simulink model "SimCases"  (R2018a)
settings: Solver=FixedStepDiscrete  StartTime=0.0  StopTime=inf  RelTol=1e-3
values from neighbouring files (symbols this model uses):
  Batch = 10    [Main.m]    (also in main.m)
  G_in = [AmbInfo(i,5,2) AmbInfo(i,:,2)]'    [Main.m]    (also in main.m)
  T_in = [AmbInfo(i,5,1) AmbInfo(i,:,1)]'    [Main.m]    (also in main.m)
libraries: dspindex x2, powerlib x1
settings Model: Creator=MATLAB  LastModifiedBy=Clayt-ML
settings OptimizationCC: SimCompilerOptimization=on
settings SFSimCC: SimParseCustomCode=off

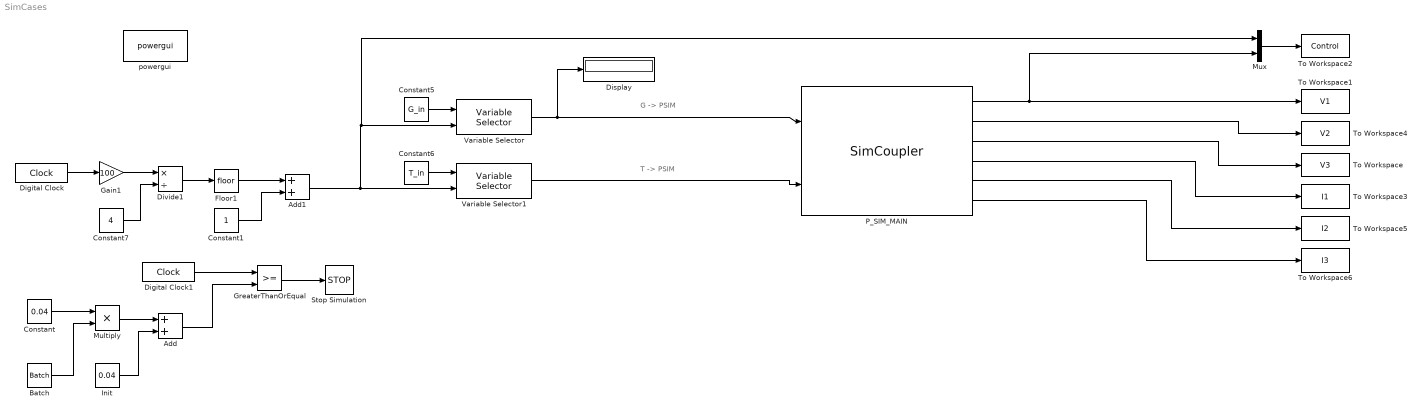
== system SimCases ==
  note: G -> PSIM
  note: T -> PSIM
  Add : Sum
  Add1 : Sum
  Batch : Constant  Value=Batch
  Constant : Constant  Value=0.04
  Constant1 : Constant
  Constant5 : Constant  Value=G_in
  Constant6 : Constant  Value=T_in
  Constant7 : Constant  Value=4
  Digital Clock : DigitalClock  SampleTime=2e-5
  Digital Clock1 : DigitalClock  SampleTime=4e-4
  Display : Display
  Divide1 : Product  Inputs=*/
  Floor1 : Rounding
  Gain1 : Gain  Gain=100
  GreaterThanOrEqual : RelationalOperator  OutDataTypeStr=boolean  RndMeth=Simplest
  Init : Constant  Value=0.04
  Multiply : Product
  Mux : Mux  Inputs=2
  P_SIM_MAIN : S-Function  FunctionName=SimCoupler  Parameters='C:\Users\Clayt-ML\Desktop\SIMUs\___Mono-Fault___02-25\S1-Normal\P_SIM_MAIN.psimsch'  SFunctionDeploymentMode=off  EnableBusSupport=off
      mask init:
      | c=[0:10:360]*pi/180;
      | x1=cos(c)*30; y1=sin(c)*30+20;
      | x2=cos(c)*30;y2=sin(c)*30-20;
      settings: OpenFcn=PsimDialog('PSimFileEdt','Value','Parameters');  CloseFcn=close(gcf);
      mask Display: plot(-60,-60,60,60,x1,y1,x2,y2)
  Stop Simulation : Stop
  To Workspace : ToWorkspace  VariableName=V3  SampleTime=-1
  To Workspace1 : ToWorkspace  VariableName=V1  SampleTime=-1
  To Workspace2 : ToWorkspace  VariableName=Control  SampleTime=-1
  To Workspace3 : ToWorkspace  VariableName=I1  SampleTime=-1
  To Workspace4 : ToWorkspace  VariableName=V2  SampleTime=-1
  To Workspace5 : ToWorkspace  VariableName=I2  SampleTime=-1
  To Workspace6 : ToWorkspace  VariableName=I3  SampleTime=-1
  Variable Selector : dspindex/Variable Selector  NumInputs=1  rowsOrCols=Rows  IdxMode=Variable  Elements=[1 3]  ZerOneIdxMode=One-based  errmode=Clip Index  FillMode=on  FillValues=0
  Variable Selector1 : dspindex/Variable Selector  NumInputs=1  rowsOrCols=Rows  IdxMode=Variable  Elements=[1 3]  ZerOneIdxMode=One-based  errmode=Clip Index  FillMode=on  FillValues=0
  powergui : powerlib/powergui  Priority=1  SimulationMode=Discrete  SampleTime=1e-5  frequency=60  Iterations=50  frequencyindice=60  Pbase=100e6  ErrMax=1e-4  UnitsV=kV  UnitsW=MW  buscounter=0  FunctionMessages=off  echomessages=off  EnableUseOfTLC=off  CurrentSourceSwitches=off  DisableSnubberDevices=off  DisableRonSwitches=off  DisableVfSwitches=off  DisplayEquations=off  SolverType=Tustin/Backward Euler (TBE)  Interpol=off  ExternalGateDelay=off  methode=off  Ts=100  x0status=blocks  SPID=on  SwTol=0  HookPort=off  RestoreLinks=warning  ResistiveCurrentMeasurement=off  Frange=[0:2:500]  Ylog=off  Xlog=on  ShowGrid=off  save=off  variable=ZData  structure=0  ZoomFFT=off  StartTime=0.0  cycles=1  DisplayStyle=1  fundamental=60  FreqAxis=off  MaxFrequency=1000  frequencyindicesteady=1  RmsSteady=1  display=off
  wires:
  Mux/1 -> To Workspace2/1
  Constant5/1 -> Variable Selector/1
  Constant6/1 -> Variable Selector1/1
  Divide1/1 -> Floor1/1
  Gain1/1 -> Divide1/1
  Constant7/1 -> Divide1/2
  P_SIM_MAIN/1 -> Mux/2, To Workspace1/1
  GreaterThanOrEqual/1 -> Stop Simulation/1
  Add/1 -> GreaterThanOrEqual/2
  Init/1 -> Add/2
  Constant/1 -> Multiply/1
  Batch/1 -> Multiply/2
  Digital Clock/1 -> Gain1/1
  Multiply/1 -> Add/1
  Variable Selector/1 -> P_SIM_MAIN/1, Display/1
  Digital Clock1/1 -> GreaterThanOrEqual/1
  Floor1/1 -> Add1/1
  Constant1/1 -> Add1/2
  Add1/1 -> Variable Selector1/2, Mux/1, Variable Selector/2
  Variable Selector1/1 -> P_SIM_MAIN/2
  P_SIM_MAIN/2 -> To Workspace4/1
  P_SIM_MAIN/3 -> To Workspace/1
  P_SIM_MAIN/4 -> To Workspace3/1
  P_SIM_MAIN/5 -> To Workspace5/1
  P_SIM_MAIN/6 -> To Workspace6/1
